simulink library "Qinverse"  (R2014b)
settings: Solver=ode45  StartTime=0.0  StopTime=10.0  RelTol=1e-3
settings Model: Creator=Hp  LastModifiedBy=Hp

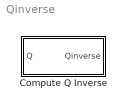
== system Qinverse ==
  Compute Q Inverse : Subsystem

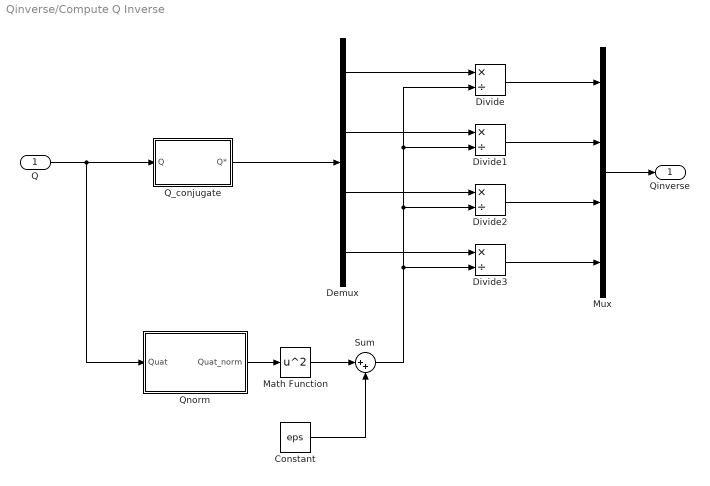
== system Qinverse/Compute Q Inverse ==
  Q : Inport
  Constant : Constant  Value=eps
  Demux : Demux
  Divide{,1..3} (4 alike) : Product  Inputs=*/
  Math Function : Math  Operator=square  SaturateOnIntegerOverflow=on
  Mux : Mux
  Q_conjugate : Subsystem
  Qnorm : Subsystem
  Sum : Sum  Inputs=|++
  Qinverse : Outport
  wires:
  Demux/3 -> Divide2/1
  Demux/1 -> Divide/1
  Qnorm/1(Quat_norm) -> Math Function/1
  Demux/4 -> Divide3/1
  Q/1 -> Qnorm/1(Quat), Q_conjugate/1(Q)
  Divide3/1 -> Mux/4
  Divide1/1 -> Mux/2
  Divide/1 -> Mux/1
  Q_conjugate/1(Q*) -> Demux/1
  Divide2/1 -> Mux/3
  Demux/2 -> Divide1/1
  Mux/1 -> Qinverse/1
  Sum/1 -> Divide3/2, Divide2/2, Divide1/2, Divide/2
  Math Function/1 -> Sum/1
  Constant/1 -> Sum/2

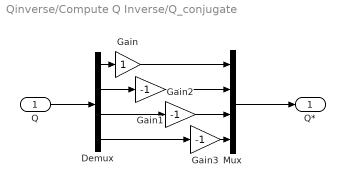
== system Qinverse/Compute Q Inverse/Q_conjugate ==
  Q : Inport
  Demux : Demux
  Gain : Gain
  Gain1 : Gain  Gain=-1
  Gain2 : Gain  Gain=-1
  Gain3 : Gain  Gain=-1
  Mux : Mux
  Q* : Outport
  wires:
  Demux/1 -> Gain/1
  Gain/1 -> Mux/1
  Mux/1 -> Q*/1
  Demux/4 -> Gain3/1
  Gain1/1 -> Mux/2
  Demux/3 -> Gain2/1
  Demux/2 -> Gain1/1
  Gain2/1 -> Mux/3
  Q/1 -> Demux/1
  Gain3/1 -> Mux/4

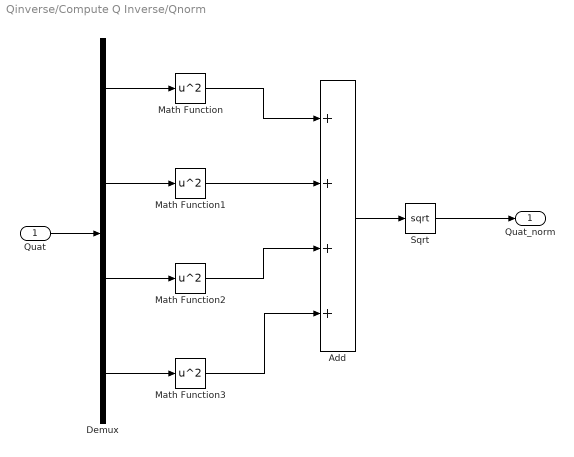
== system Qinverse/Compute Q Inverse/Qnorm ==
  Quat : Inport
  Add : Sum  Inputs=++++
  Demux : Demux
  Math Function{,1..3} (4 alike) : Math  Operator=square  SaturateOnIntegerOverflow=on
  Sqrt : Sqrt  SaturateOnIntegerOverflow=on
  Quat_norm : Outport
  wires:
  Math Function2/1 -> Add/3
  Math Function/1 -> Add/1
  Add/1 -> Sqrt/1
  Math Function3/1 -> Add/4
  Math Function1/1 -> Add/2
  Demux/3 -> Math Function2/1
  Demux/1 -> Math Function/1
  Demux/4 -> Math Function3/1
  Sqrt/1 -> Quat_norm/1
  Demux/2 -> Math Function1/1
  Quat/1 -> Demux/1
